simulink model "ssc_lithium_cell_1RC_estim"  (Simulink 7.6)
settings: Solver=ode15s  StartTime=0  StopTime=37000  MaxStep=250  RelTol=1e-3
PreLoadFcn:
  | ssc_lithium_cell_1RC_estim_ini
libraries: fl_lib x8, LiBatteryElements_lib x4, nesl_utility x4
settings Model: Creator=psanghvi  LastModifiedBy=rjackey
settings DataIOCC: ExternalInput=[PulseData.time PulseData.current PulseData.voltage]  LimitDataPoints=off  LoadExternalInput=on  SignalLogging=off  DSMLogging=off
settings OptimizationCC: EnhancedBackFolding=on  OptimizeModelRefInitCode=on  LifeSpan=1  SimCompilerOptimization=On
settings RTWCC: SystemTargetFile=ert.tlc  GenCodeOnly=on  TemplateMakefile=ert_default_tmf  Description=Embedded Coder  GenerateReport=on  ProcessScript=ert_make_rtw_hook  IncludeHyperlinkInReport=on  LaunchReport=on  GenerateTraceInfo=on  GenerateTraceReport=on  GenerateTraceReportSl=on  GenerateTraceReportSf=on  GenerateTraceReportEml=on
settings CodeAppCC: IgnoreCustomStorageClasses=off
settings ERTTargetCC: MultiwordLength=2048  GenerateSampleERTMain=on  ERTCustomFileTemplate=example_file_process.tlc  ConvertIfToSwitch=off

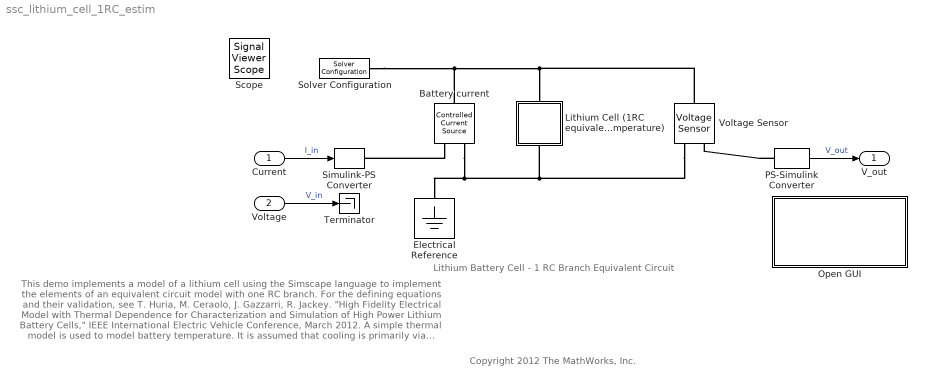
== system ssc_lithium_cell_1RC_estim ==
  note: Lithium Battery Cell - 1 RC Branch Equivalent Circuit
  note: This demo implements a model of a lithium cell using the Simscape language to implement the elements of an equivalent circuit model with one
      | RC branch. For the defining equations and their validation, see T. Huria, M. Ceraolo, J. Gazzarri, R. Jackey. "High Fidelity Electrical Model with
      | Thermal Dependence for Characterization and Simulation of High Power Lithium Battery Cells," IEEE International Electric Vehicle Conference,
      | March 2012. A simple thermal model is used to model battery temperature. It is assumed that cooling is primarily via convection, and that heating
      | is primarily from internal resistance. A battery pack can be modeled by connecting multiple copies of the battery cell block in series.
  note: Copyright 2012 The MathWorks, Inc.
  Current : Inport
  Voltage : Inport  Port=2
  Battery current : fl_lib/Electrical/Electrical Sources/Controlled Current Source  DialogController=NetworkEngine.DynNeDlgSource  SystemSampleTime=-1  i_Log=off  v_Log=off  LocalVarNames=|current|voltage|power  LocalVarDescs=|Current (A)|Voltage (V)|Power (W)  LocalVarLogging=[0 0 0]
  Electrical Reference : fl_lib/Electrical/Electrical Elements/Electrical Reference  DialogController=NetworkEngine.DynNeDlgSource  SystemSampleTime=-1  i_Log=off  LocalVarNames=|i  LocalVarDescs=|i  LocalVarLogging=[]
  "Lithium Cell (1RC equivalent circuit model,  single temperature)" : Subsystem
  Open GUI : Subsystem
      settings: OpenFcn=speload('ssc_lithium_cell_SDO_Project', 'Project - ssc_lithium_cell_1RC_estim', 'One Temp Estim');
      mask Display: disp('Double click here\nto open the\nParameter Estimation\nGUI with preloaded data')
  PS-Simulink Converter : nesl_utility/PS-Simulink Converter  DialogController=NetworkEngine.DynNeUtilDlgSource  SystemSampleTime=-1  PhysicalDomain=network_engine_domain  LeftPortType=input  RightPortType=output  SubClassName=ps_output  Unit=V  AffineConversion=off
  Simulink-PS Converter : nesl_utility/Simulink-PS Converter  DialogController=NetworkEngine.DynNeUtilDlgSource  SystemSampleTime=-1  PhysicalDomain=network_engine_domain  LeftPortType=input  RightPortType=output  SubClassName=ps_input  Unit=A  AffineConversion=off  InputFilterTimeConstant=.001  UdotUserProvided=0
  Solver Configuration : nesl_utility/Solver Configuration  DialogController=NetworkEngine.DynNeUtilDlgSource  SystemSampleTime=-1  PhysicalDomain=network_engine_domain  LeftPortType=input  RightPortType=generic  SubClassName=solver  Accelerate=off  Profile=off  ResidualTolerance=1e-9  MaxNonlinIter=12  MaxModeIter=2  DoFixedCost=off  UseLocalSampling=off  DoDC=off  LinearAlgebra=Sparse  LocalSolverSampleTime=.001  LocalSolverChoice=NE_BACKWARD_EULER_ADVANCER  UseLocalSolver=off
  Terminator : Terminator
  Voltage Sensor : fl_lib/Electrical/Electrical Sensors/Voltage Sensor  DialogController=NetworkEngine.DynNeDlgSource  SystemSampleTime=-1  i1_Log=off  v1_Log=off  LocalVarNames=|i1|v1  LocalVarDescs=|i1|v1  LocalVarLogging=[]
  V_out : Outport
  Scope : SignalViewerScope  IOType=viewer  NumInputPorts=3  RefreshTime=0.035000
      settings: TimeRange=40000  YMin=3.15~-30~0  YMax=4.25~2~1
  wires:
  PS-Simulink Converter/1 -> V_out/1  "V_out"
  Current/1 -> Simulink-PS Converter/1  "I_in"
  Voltage/1 -> Terminator/1  "V_in"
  connections:
  Battery current/RConn1 -- Simulink-PS Converter/RConn1
  Battery current/LConn1 -- "Lithium Cell (1RC equivalent circuit model,  single temperature)"/LConn1 -- Voltage Sensor/LConn1 -- Solver Configuration/RConn1
  PS-Simulink Converter/LConn1 -- Voltage Sensor/RConn1
  Voltage Sensor/RConn2 -- "Lithium Cell (1RC equivalent circuit model,  single temperature)"/RConn1 -- Battery current/RConn2 -- Electrical Reference/LConn1

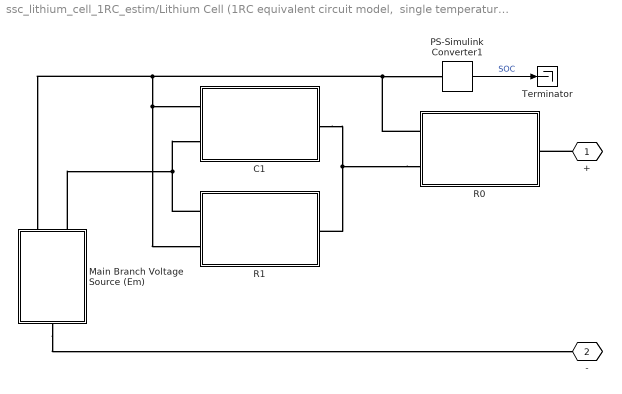
== system ssc_lithium_cell_1RC_estim/Lithium Cell (1RC equivalent circuit model,  single temperature) ==
  C1 : Subsystem
  Main Branch Voltage Source (Em) : Subsystem
  PS-Simulink Converter1 : nesl_utility/PS-Simulink Converter  DialogController=NetworkEngine.DynNeUtilDlgSource  SystemSampleTime=-1  PhysicalDomain=network_engine_domain  LeftPortType=input  RightPortType=output  SubClassName=ps_output  Unit=1  AffineConversion=off
  R0 : Subsystem
  R1 : Subsystem
  Terminator : Terminator
  + : PMIOPort  Tag=PMCPort  Port=1  Side=Left
  - : PMIOPort  Tag=PMCPort  Port=2  Side=Right
  wires:
  PS-Simulink Converter1/1 -> Terminator/1  "SOC"
  connections:
  R1/LConn1 -- Main Branch Voltage Source (Em)/LConn2 -- C1/LConn2
  +/RConn1 -- R0/RConn1
  Main Branch Voltage Source (Em)/RConn1 -- -/RConn1
  R0/LConn1 -- C1/LConn1 -- R1/LConn2 -- Main Branch Voltage Source (Em)/LConn1 -- PS-Simulink Converter1/LConn1
  R0/LConn2 -- C1/RConn1 -- R1/RConn1

== system ssc_lithium_cell_1RC_estim/Open GUI ==

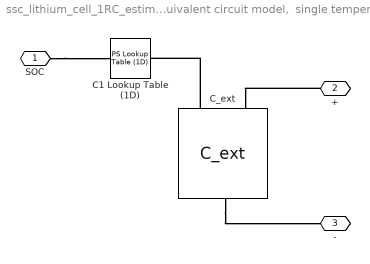
== system ssc_lithium_cell_1RC_estim/Lithium Cell (1RC equivalent circuit model,  single temperature)/C1 ==
  C1 Lookup Table (1D) : fl_lib/Physical Signals/Lookup Tables/PS Lookup Table (1D)  DialogController=NetworkEngine.DynNeDlgSource  SystemSampleTime=-1  x_t=SOC_LUT  y_t=C1  interp_method=1  extrap_method=1  dbg=0  LocalVarLogging=[]
  C_ext : LiBatteryElements_lib/C_ext  DialogController=NetworkEngine.DynNeDlgSource  SystemSampleTime=-1  v0=0 V  Cmin=1e-6 F  i_Log=off  v_Log=off  LocalVarNames=|i|v  LocalVarDescs=|i|v  LocalVarLogging=[0 0]
  SOC : PMIOPort  Port=1  Side=Left
  + : PMIOPort  Port=2  Side=Left
  - : PMIOPort  Port=3  Side=Right
  connections:
  +/RConn1 -- C_ext/LConn1
  C_ext/RConn1 -- -/RConn1
  C_ext/LConn2 -- C1 Lookup Table (1D)/RConn1
  SOC/RConn1 -- C1 Lookup Table (1D)/LConn1

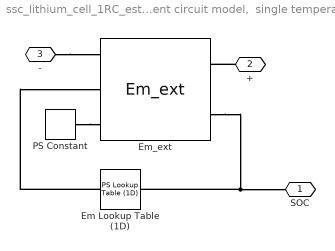
== system ssc_lithium_cell_1RC_estim/Lithium Cell (1RC equivalent circuit model,  single temperature)/Main Branch Voltage Source (Em) ==
  Em Lookup Table (1D) : fl_lib/Physical Signals/Lookup Tables/PS Lookup Table (1D)  DialogController=NetworkEngine.DynNeDlgSource  SystemSampleTime=-1  x_t=SOC_LUT  y_t=Em  interp_method=1  extrap_method=1  dbg=0  LocalVarLogging=[]
  Em_ext : LiBatteryElements_lib/Em_ext  DialogController=NetworkEngine.DynNeDlgSource  SystemSampleTime=-1  Qinit=Qe_init hr*A  i_Log=off  v_Log=off  Qe_Log=off  LocalVarNames=|i|v|Qe  LocalVarDescs=|i|v|Extracted charge  LocalVarLogging=[0 0 0]
  PS Constant : fl_lib/Physical Signals/Sources/PS Constant  DialogController=NetworkEngine.DynNeDlgSource  SystemSampleTime=-1  constant=Capacity  LocalVarLogging=[]
  SOC : PMIOPort  Port=1  Side=Left
  + : PMIOPort  Port=2  Side=Left
  - : PMIOPort  Port=3  Side=Right
  connections:
  Em_ext/LConn2 -- SOC/RConn1 -- Em Lookup Table (1D)/LConn1
  +/RConn1 -- Em_ext/LConn1
  -/RConn1 -- Em_ext/RConn1
  Em Lookup Table (1D)/RConn1 -- Em_ext/RConn2
  PS Constant/RConn1 -- Em_ext/RConn3

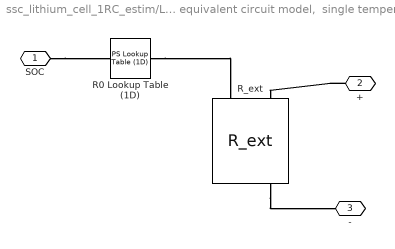
== system ssc_lithium_cell_1RC_estim/Lithium Cell (1RC equivalent circuit model,  single temperature)/R0 ==
  R0 Lookup Table (1D) : fl_lib/Physical Signals/Lookup Tables/PS Lookup Table (1D)  DialogController=NetworkEngine.DynNeDlgSource  SystemSampleTime=-1  x_t=SOC_LUT  y_t=R0  interp_method=1  extrap_method=1  dbg=0  LocalVarLogging=[]
  R_ext : LiBatteryElements_lib/R_ext  DialogController=NetworkEngine.DynNeDlgSource  SystemSampleTime=-1  Rmin=0 Ohm  i_Log=off  v_Log=off  LocalVarNames=|i|v  LocalVarDescs=|i|v  LocalVarLogging=[0 0]
  SOC : PMIOPort  Port=1  Side=Left
  + : PMIOPort  Port=2  Side=Left
  - : PMIOPort  Port=3  Side=Right
  connections:
  SOC/RConn1 -- R0 Lookup Table (1D)/LConn1
  R0 Lookup Table (1D)/RConn1 -- R_ext/LConn2
  R_ext/RConn1 -- -/RConn1
  +/RConn1 -- R_ext/LConn1

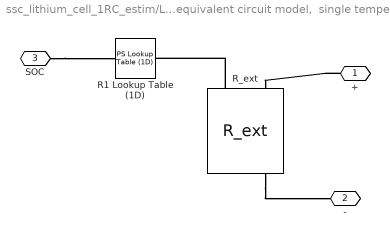
== system ssc_lithium_cell_1RC_estim/Lithium Cell (1RC equivalent circuit model,  single temperature)/R1 ==
  R1 Lookup Table (1D) : fl_lib/Physical Signals/Lookup Tables/PS Lookup Table (1D)  DialogController=NetworkEngine.DynNeDlgSource  SystemSampleTime=-1  x_t=SOC_LUT  y_t=R1  interp_method=1  extrap_method=1  dbg=0  LocalVarLogging=[]
  R_ext : LiBatteryElements_lib/R_ext  DialogController=NetworkEngine.DynNeDlgSource  SystemSampleTime=-1  Rmin=0 Ohm  i_Log=off  v_Log=off  LocalVarNames=|i|v  LocalVarDescs=|i|v  LocalVarLogging=[0 0]
  + : PMIOPort  Port=1  Side=Left
  - : PMIOPort  Port=2  Side=Right
  SOC : PMIOPort  Port=3  Side=Left
  connections:
  +/RConn1 -- R_ext/LConn1
  R_ext/RConn1 -- -/RConn1
  R_ext/LConn2 -- R1 Lookup Table (1D)/RConn1
  SOC/RConn1 -- R1 Lookup Table (1D)/LConn1
